simulink model "hw3_mdkhan"  (R2017b)
settings: Solver=ode23tb  StartTime=0.0  StopTime=40  RelTol=1e-3  EnableMultiTasking=on
undefined symbols (not defined in the file): sigbuilder_block
libraries: simulink x1
settings Model: Creator=sampad  LastModifiedBy=khan1
settings DataIOCC: LimitDataPoints=on
settings OptimizationCC: LifeSpan=inf
settings DebuggingCC: AllowSymbolicDim=off  SFUnexpectedBacktrackingDiag=warning  SFNoUnconditionalDefaultTransitionDiag=warning  SFExecutionAtInitializationDiag=none
settings ModelReferenceCC: PropagateSignalLabelsOutOfModel=off
settings CodeAppCC: StateflowObjectComments=on
settings GRTTargetCC: TargetLangStandard=C89/C90 (ANSI)
settings ConfigComp: CovMetricSettings=dw  CovHTMLOptions=-sRT=1 -sVT=0 -aTS=1 -bRG=1 -bTC=1 -hTR=0 -nFC=0 -nFD=1 -scm=1 -bcm=1 -xEv=0 -xEM=0  CovHtmlReporting=on  CovSaveCumulativeToWorkspaceVar=on  CovSaveSingleToWorkspaceVar=on  CovExternalEMLEnable=off

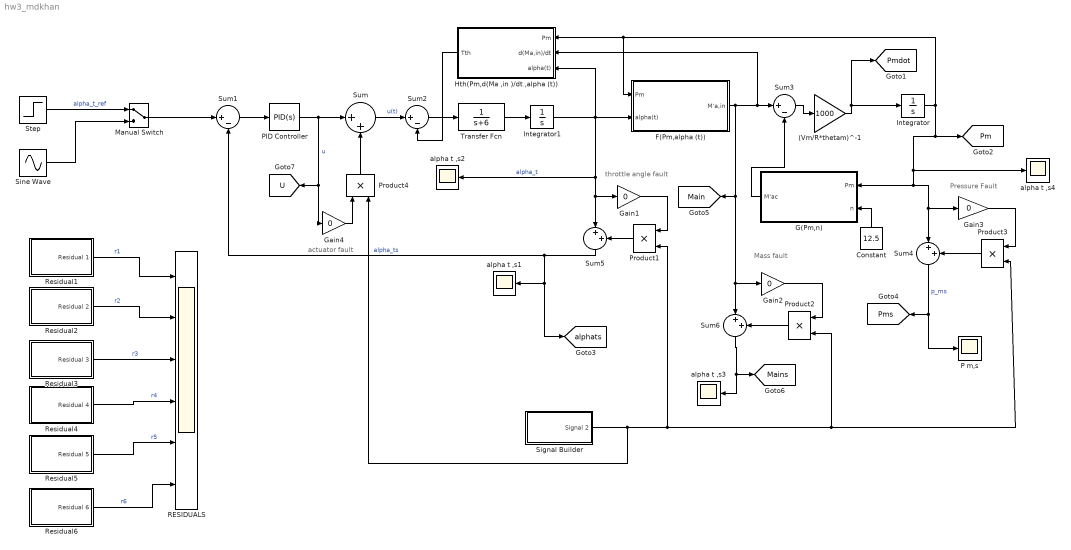
== system hw3_mdkhan ==
  note: actuator fault
  note: throttle angle fault
  note: Mass fault
  note: Pressure Fault
  (Vm/R*thetam)^-1 : Gain  Gain=1000
  Constant : Constant  Value=12.5
  F(Pm,alpha (t)) : Subsystem
  G(Pm,n) : Subsystem
  Gain{1..4} (4 alike) : Gain  Gain=0
  Hth(Pm,d(Ma ,in )/dt ,alpha (t)) : Subsystem
  Integrator : Integrator
  Integrator1 : Integrator
  Manual Switch : ManualSwitch
  P m,s : Scope
  PID Controller : simulink/Continuous/PID Controller  Controller=PID  TimeDomain=Continuous-time  SampleTime=-1  IntegratorMethod=Forward Euler  FilterMethod=Forward Euler  Form=Parallel  UseFilter=on  ControllerParametersSource=internal  P=50.7443606620062  I=163.284224308189  D=3.90171175948325  N=829.275839878731  InitialConditionSource=internal  InitialConditionForIntegrator=0  InitialConditionForFilter=0  ExternalReset=none  LimitOutput=off  UpperSaturationLimit=inf  LowerSaturationLimit=-inf  LinearizeAsGain=on  AntiWindupMode=none  Kb=1  TrackingMode=off  Kt=1  PParamMin=[]  PParamMax=[]  IParamMin=[]  IParamMax=[]  DParamMin=[]  DParamMax=[]  NParamMin=[]  NParamMax=[]  KbParamMin=[]  KbParamMax=[]  KtParamMin=[]  KtParamMax=[]  POutMin=[]  POutMax=[]  IOutMin=[]  IOutMax=[]  DOutMin=[]  DOutMax=[]  NOutMin=[]  NOutMax=[]  KbOutMin=[]  KbOutMax=[]  KtOutMin=[]  KtOutMax=[]  IntegratorOutMin=[]  IntegratorOutMax=[]  FilterOutMin=[]  FilterOutMax=[]  SumOutMin=[]  SumOutMax=[]  SumI1OutMin=[]  SumI1OutMax=[]  SumI2OutMin=[]  SumI2OutMax=[]  SumI3OutMin=[]  SumI3OutMax=[]  SumDOutMin=[]  SumDOutMax=[]  SaturationOutMin=[]  SaturationOutMax=[]  IntegratorContinuousStateAttributes=''  IntegratorStateMustResolveToSignalObject=off  IntegratorRTWStateStorageClass=Auto  FilterContinuousStateAttributes=''  FilterStateMustResolveToSignalObject=off  FilterRTWStateStorageClass=Auto  DifferentiatorICPrevScaledInput=0  DifferentiatorOutMin=[]  DifferentiatorOutMax=[]  InitialConditionSetting=State (most efficient)  FilterDiffOutCoefMin=[]  FilterDiffOutCoefMax=[]  SumDenOutMin=[]  SumDenOutMax=[]  SumNumOutMin=[]  SumNumOutMax=[]  ReciprocalOutMin=[]  ReciprocalOutMax=[]  DivideOutMin=[]  DivideOutMax=[]  TunerSelectOption=Transfer Function Based (PID Tuner App)
  Product{1..4} (4 alike) : Product  RndMeth=Zero
  RESIDUALS : Scope  NumInputPorts=6
  Residual1 : Subsystem
  Residual2 : Subsystem
  Residual3 : Subsystem
  Residual4 : Subsystem
  Residual5 : Subsystem
  Residual6 : Subsystem
  Signal Builder : Subsystem  Tag=STV Subsys  LoadFcn=sigbuilder_block('load');  StartFcn=sigbuilder_block('start');  StopFcn=sigbuilder_block('stop');  ClipboardFcn=sigbuilder_block('clipboard');  mask(Sigbuilder block){tuvar=[0:10]}
      mask help: Create and generate interchangeable groups of signals whose waveforms are piecewise linear.
      mask init:
      | if ~strcmp(get_param(bdroot(gcbh),'SimulationStatus'),'stopped') tuvar = sigbuilder_block('maskInit'); end
      settings: CopyFcn=sigbuilder_block('copy');  DeleteFcn=sigbuilder_block('delete');  ModelCloseFcn=sigbuilder_block('modelClose');  PreSaveFcn=sigbuilder_block('preSave');  PauseFcn=sigbuilder_block('pause')  ContinueFcn=sigbuilder_block('continue')  NameChangeFcn=sigbuilder_block('namechange');  OpenFcn=sigbuilder_block('open',[437.25 117.75 550.5 394.5 ]);  CloseFcn=sigbuilder_block('close');
      mask Display: plot(0, 0, 100, 100,[2, 2, 32, 32, 2], [68, 8, 8, 68, 68],[32, 2], [38, 38], [32, 19, 2],[53, 60, 44], [32, 17, 17, 2],[16, 16, 31, 31]);txt = getActiveGroup(gcbh);text(2, 100, txt,'verticalAlignment', 'top');
  Sine Wave : Sin  SampleTime=0
  Step : Step  Time=0.01  After=20  SampleTime=0
  Sum : Sum  Inputs=|++
  Sum1 : Sum  Inputs=|+-
  Sum2 : Sum  Inputs=|+-
  Sum3 : Sum  Inputs=|+-
  Sum4 : Sum  Inputs=|++  CollapseMode=Specified dimension
  Sum5 : Sum  Inputs=|++  CollapseMode=Specified dimension
  Sum6 : Sum  Inputs=|++  CollapseMode=Specified dimension
  Transfer Fcn : TransferFcn  Denominator=[1 6]
  alpha t ,s{1..4} (4 alike) : Scope
  tag scope: Main=global, Mains=global, Pm=global, Pmdot=global, Pms=global, U=global, alphats=global
  wires:
  Sum1/1 -> PID Controller/1
  PID Controller/1 -> Gain4/1, [U], Sum/1  "u"
  Sum/1 -> Sum2/1  "u(t)"
  Sum2/1 -> Transfer Fcn/1
  Integrator1/1 -> alpha t ,s2/1, Gain1/1, Sum5/1, F(Pm,alpha (t))/2(alpha(t)), Hth(Pm,d(Ma ,in )/dt ,alpha (t))/3(alpha(t))  "alpha_t"
  (Vm/R*thetam)^-1/1 -> Integrator/1, [Pmdot]
  Sum3/1 -> (Vm/R*thetam)^-1/1
  Hth(Pm,d(Ma ,in )/dt ,alpha (t))/1(Tth) -> Sum2/2
  Transfer Fcn/1 -> Integrator1/1
  Product1/1 -> Sum5/2
  Gain1/1 -> Product1/1
  F(Pm,alpha (t))/1(M'a,in) -> [Main], Gain2/1, Sum6/1, Hth(Pm,d(Ma ,in )/dt ,alpha (t))/2(d(Ma,in)/dt), Sum3/1
  Product2/1 -> Sum6/2
  Sum6/1 -> alpha t ,s3/1, [Mains]
  G(Pm,n)/1(M'ac) -> Sum3/2
  Integrator/1 -> F(Pm,alpha (t))/1(Pm), Hth(Pm,d(Ma ,in )/dt ,alpha (t))/1(Pm), alpha t ,s4/1, Gain3/1, Sum4/1, G(Pm,n)/1(Pm), [Pm]
  Product3/1 -> Sum4/2
  Gain3/1 -> Product3/1
  Residual1/1(Residual 1) -> RESIDUALS/1  "r1"
  Residual2/1(Residual 2) -> RESIDUALS/2  "r2"
  Residual3/1(Residual 3) -> RESIDUALS/3  "r3"
  Residual4/1(Residual 4) -> RESIDUALS/4  "r4"
  Residual5/1(Residual 5) -> RESIDUALS/5  "r5"
  Residual6/1(Residual 6) -> RESIDUALS/6  "r6"
  Step/1 -> Manual Switch/1  "alpha_t_ref"
  Manual Switch/1 -> Sum1/1
  Sine Wave/1 -> Manual Switch/2
  Sum5/1 -> [alphats], alpha t ,s1/1, Sum1/2  "alpha_ts"
  Gain2/1 -> Product2/1
  Constant/1 -> G(Pm,n)/2(n)
  Sum4/1 -> P m,s/1, [Pms]  "p_ms"
  Gain4/1 -> Product4/1
  Product4/1 -> Sum/2
  Signal Builder/1(Signal 2) -> Product4/2, Product3/2, Product2/2, Product1/2

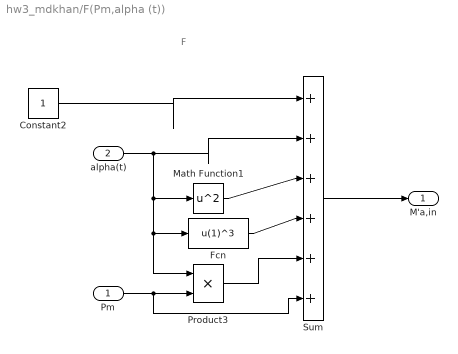
== system hw3_mdkhan/F(Pm,alpha (t)) ==
  note: F
  Pm : Inport
  alpha(t) : Inport  Port=2
  Constant2 : Constant
  Fcn : Fcn  Expr=u(1)^3
  Math Function1 : Math  Operator=square  SaturateOnIntegerOverflow=on
  Product3 : Product  RndMeth=Zero
  Sum : Sum  Inputs=|++++++
  M'a,in : Outport
  wires:
  Sum/1 -> M'a,in/1
  Constant2/1 -> Sum/1
  alpha(t)/1 -> Sum/2, Math Function1/1, Fcn/1, Product3/1
  Math Function1/1 -> Sum/3
  Fcn/1 -> Sum/4
  Product3/1 -> Sum/5
  Pm/1 -> Product3/2, Sum/6

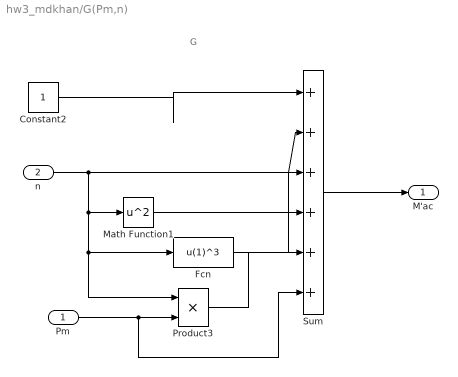
== system hw3_mdkhan/G(Pm,n) ==
  note: G
  Pm : Inport
  n : Inport  Port=2
  Constant2 : Constant
  Fcn : Fcn  Expr=u(1)^3
  Math Function1 : Math  Operator=square  SaturateOnIntegerOverflow=on
  Product3 : Product  RndMeth=Zero
  Sum : Sum  Inputs=|++++++
  M'ac : Outport
  wires:
  Sum/1 -> M'ac/1
  Constant2/1 -> Sum/1
  n/1 -> Sum/2, Math Function1/1, Fcn/1, Product3/1
  Math Function1/1 -> Sum/3
  Fcn/1 -> Sum/4
  Pm/1 -> Product3/2, Sum/6
  Product3/1 -> Sum/5

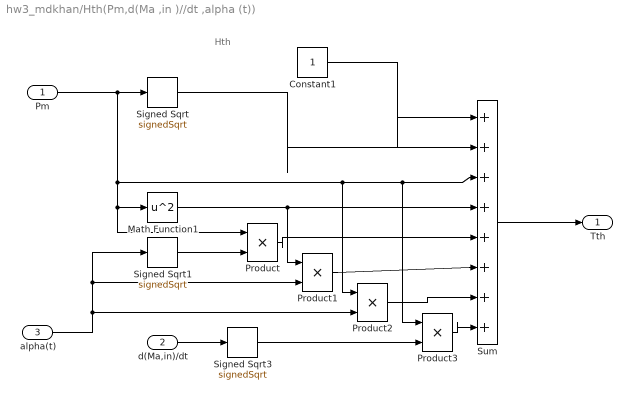
== system hw3_mdkhan/Hth(Pm,d(Ma ,in )//dt ,alpha (t)) ==
  note: Hth
  Pm : Inport
  d(Ma,in)/dt : Inport  Port=2
  alpha(t) : Inport  Port=3
  Constant1 : Constant
  Math Function1 : Math  Operator=square  SaturateOnIntegerOverflow=on
  Product{,1..3} (4 alike) : Product  RndMeth=Zero
  Signed Sqrt : Sqrt  Operator=signedSqrt  SaturateOnIntegerOverflow=on
  Signed Sqrt1 : Sqrt  Operator=signedSqrt  SaturateOnIntegerOverflow=on
  Signed Sqrt3 : Sqrt  Operator=signedSqrt  SaturateOnIntegerOverflow=on
  Sum : Sum  Inputs=|++++++++
  Tth : Outport
  wires:
  Constant1/1 -> Sum/1
  Pm/1 -> Signed Sqrt/1, Math Function1/1, Product/1, Product2/1, Sum/3, Product3/1
  Signed Sqrt/1 -> Sum/2
  Math Function1/1 -> Sum/4, Product1/1
  alpha(t)/1 -> Signed Sqrt1/1, Product1/2, Product2/2
  Signed Sqrt1/1 -> Product/2
  Product/1 -> Sum/5
  Product1/1 -> Sum/6
  Product2/1 -> Sum/7
  Product3/1 -> Sum/8
  d(Ma,in)/dt/1 -> Signed Sqrt3/1
  Signed Sqrt3/1 -> Product3/2
  Sum/1 -> Tth/1

== system hw3_mdkhan/Residual1 ==
  F(Pm,alpha (t)) : Subsystem
  Sum : Sum  Inputs=|+-
  Residual 1 : Outport
  wires:
  [Mains] -> Sum/1
  [Pms] -> F(Pm,alpha (t))/1(Pm)
  [alphats] -> F(Pm,alpha (t))/2(alpha(t))
  F(Pm,alpha (t))/1(M'a,in) -> Sum/2
  Sum/1 -> Residual 1/1

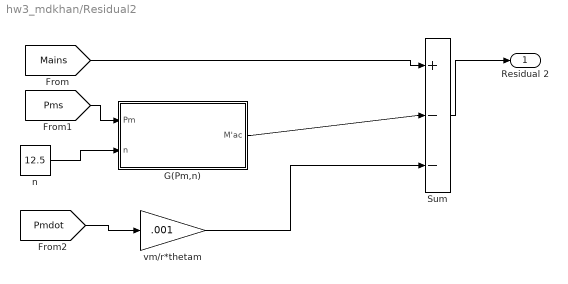
== system hw3_mdkhan/Residual2 ==
  G(Pm,n) : Subsystem
  Sum : Sum  Inputs=|+--
  n : Constant  Value=12.5
  vm/r*thetam : Gain  Gain=.001
  Residual 2 : Outport
  wires:
  Sum/1 -> Residual 2/1
  [Mains] -> Sum/1
  [Pms] -> G(Pm,n)/1(Pm)
  n/1 -> G(Pm,n)/2(n)
  G(Pm,n)/1(M'ac) -> Sum/2
  [Pmdot] -> vm/r*thetam/1
  vm/r*thetam/1 -> Sum/3

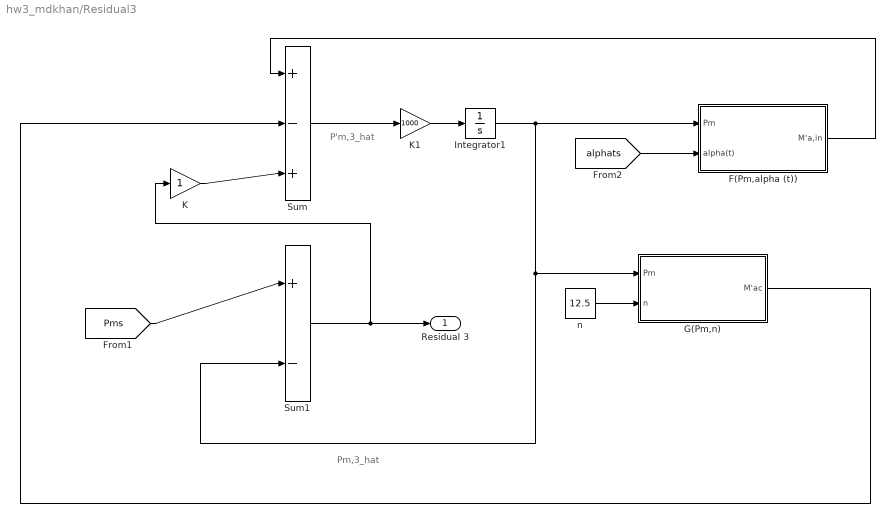
== system hw3_mdkhan/Residual3 ==
  note: Pm,3_hat
  note: P'm,3_hat
  F(Pm,alpha (t)) : Subsystem
  G(Pm,n) : Subsystem
  Integrator1 : Integrator
  K : Gain
  K1 : Gain  Gain=1000
  Sum : Sum  Inputs=|+-+
  Sum1 : Sum  Inputs=|+-
  n : Constant  Value=12.5
  Residual 3 : Outport
  wires:
  [Pms] -> Sum1/1
  K/1 -> Sum/3
  Sum1/1 -> K/1, Residual 3/1
  Sum/1 -> K1/1
  K1/1 -> Integrator1/1
  Integrator1/1 -> F(Pm,alpha (t))/1(Pm), Sum1/2, G(Pm,n)/1(Pm)
  [alphats] -> F(Pm,alpha (t))/2(alpha(t))
  F(Pm,alpha (t))/1(M'a,in) -> Sum/1
  n/1 -> G(Pm,n)/2(n)
  G(Pm,n)/1(M'ac) -> Sum/2

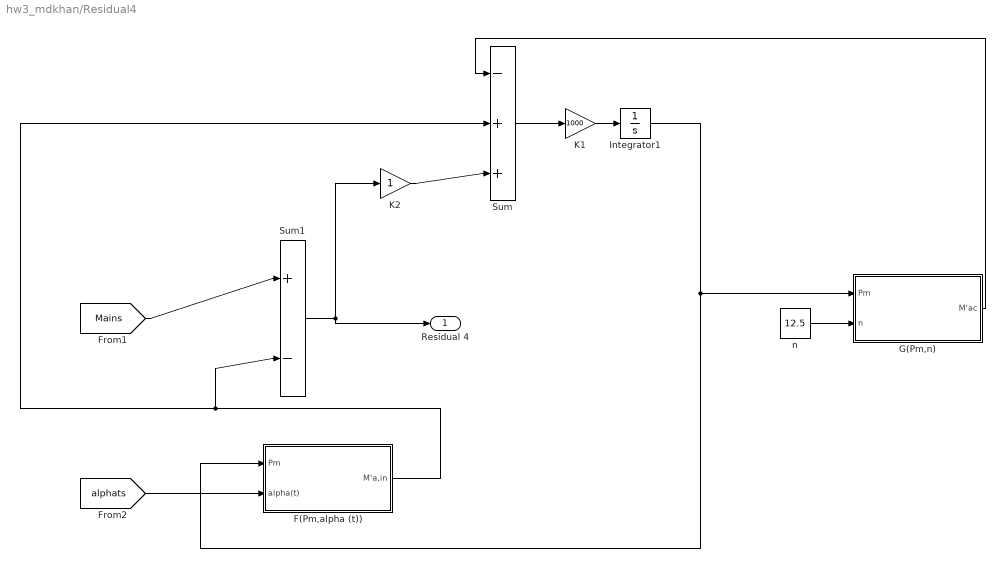
== system hw3_mdkhan/Residual4 ==
  F(Pm,alpha (t)) : Subsystem
  G(Pm,n) : Subsystem
  Integrator1 : Integrator
  K1 : Gain  Gain=1000
  K2 : Gain
  Sum : Sum  Inputs=|-++
  Sum1 : Sum  Inputs=|+-
  n : Constant  Value=12.5
  Residual 4 : Outport
  wires:
  n/1 -> G(Pm,n)/2(n)
  K1/1 -> Integrator1/1
  Sum/1 -> K1/1
  K2/1 -> Sum/3
  [Mains] -> Sum1/1
  [alphats] -> F(Pm,alpha (t))/2(alpha(t))
  Sum1/1 -> Residual 4/1, K2/1
  F(Pm,alpha (t))/1(M'a,in) -> Sum/2, Sum1/2
  Integrator1/1 -> F(Pm,alpha (t))/1(Pm), G(Pm,n)/1(Pm)
  G(Pm,n)/1(M'ac) -> Sum/1

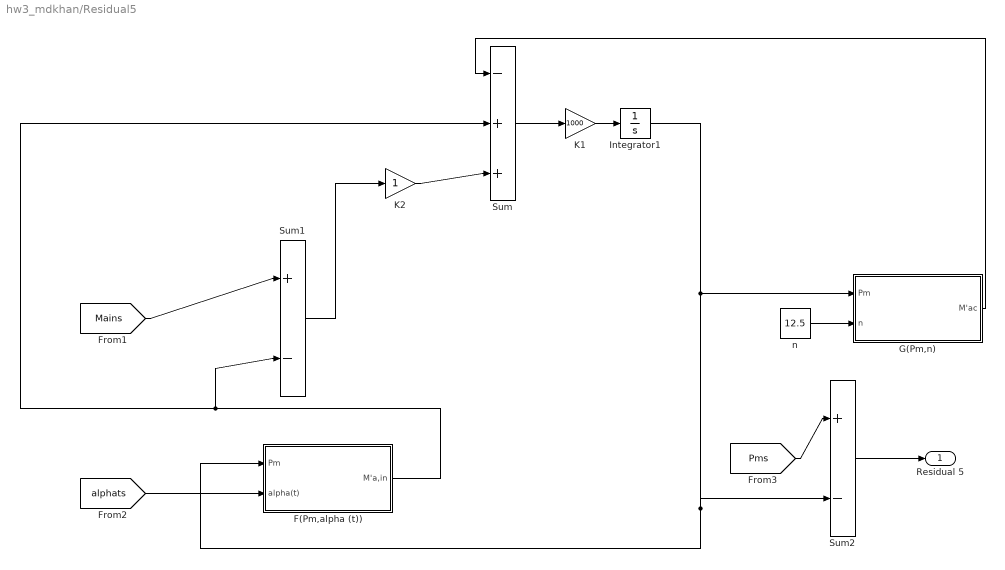
== system hw3_mdkhan/Residual5 ==
  F(Pm,alpha (t)) : Subsystem
  G(Pm,n) : Subsystem
  Integrator1 : Integrator
  K1 : Gain  Gain=1000
  K2 : Gain
  Sum : Sum  Inputs=|-++
  Sum1 : Sum  Inputs=|+-
  Sum2 : Sum  Inputs=|+-
  n : Constant  Value=12.5
  Residual 5 : Outport
  wires:
  G(Pm,n)/1(M'ac) -> Sum/1
  Integrator1/1 -> G(Pm,n)/1(Pm), F(Pm,alpha (t))/1(Pm), Sum2/2
  F(Pm,alpha (t))/1(M'a,in) -> Sum1/2, Sum/2
  Sum1/1 -> K2/1
  [alphats] -> F(Pm,alpha (t))/2(alpha(t))
  [Mains] -> Sum1/1
  K2/1 -> Sum/3
  Sum/1 -> K1/1
  K1/1 -> Integrator1/1
  n/1 -> G(Pm,n)/2(n)
  Sum2/1 -> Residual 5/1
  [Pms] -> Sum2/1

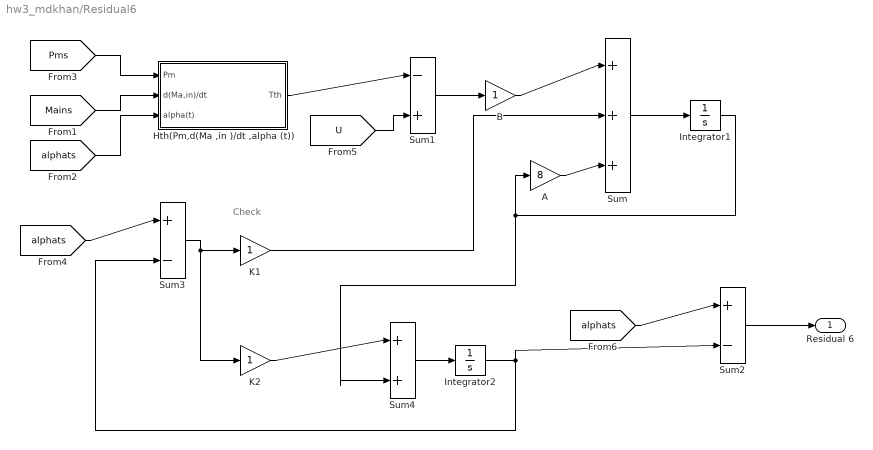
== system hw3_mdkhan/Residual6 ==
  note: Check
  A : Gain  Gain=8
  B : Gain
  Hth(Pm,d(Ma ,in )/dt ,alpha (t)) : Subsystem
  Integrator1 : Integrator
  Integrator2 : Integrator
  K1 : Gain
  K2 : Gain
  Sum : Sum  Inputs=|+++
  Sum1 : Sum  Inputs=|-+
  Sum2 : Sum  Inputs=|+-
  Sum3 : Sum  Inputs=|+-
  Sum4 : Sum  Inputs=|++
  Residual 6 : Outport
  wires:
  [Pms] -> Hth(Pm,d(Ma ,in )/dt ,alpha (t))/1(Pm)
  [Mains] -> Hth(Pm,d(Ma ,in )/dt ,alpha (t))/2(d(Ma,in)/dt)
  [alphats] -> Hth(Pm,d(Ma ,in )/dt ,alpha (t))/3(alpha(t))
  Hth(Pm,d(Ma ,in )/dt ,alpha (t))/1(Tth) -> Sum1/1
  [U] -> Sum1/2
  Sum1/1 -> B/1
  B/1 -> Sum/1
  [alphats] -> Sum3/1
  Sum3/1 -> K1/1, K2/1
  K1/1 -> Sum/2
  Sum/1 -> Integrator1/1
  Integrator1/1 -> A/1, Sum4/2
  A/1 -> Sum/3
  Sum4/1 -> Integrator2/1
  Integrator2/1 -> Sum2/2, Sum3/2
  [alphats] -> Sum2/1
  Sum2/1 -> Residual 6/1
  K2/1 -> Sum4/1

== system hw3_mdkhan/Signal Builder ==
  Demux : Demux  Tag=STV Demux  Outputs=1
  FromWs : FromWorkspace  Tag=STV FromWs  VariableName=tuvar  SampleTime=0
      SigBuilderData=|
      | common.afterFinalStr = 'Extrapolate'
      | common.sampleTime = 0
      | dataSet.timeRange = [0 50]
      | dataSet.name = 'Group 1'
      | sbobj.Groups.Name = 'Group 1'
      | sbobj.Groups.Signals.Name = 'Signal 2'
      | sbobj.Groups.Signals.XData = [0 10 10 30 30 50]
      | sbobj.Groups.Signals.YData = [0 0 1 1 0 0]
      | sbobj.Groups.TimeRange = [0 50]
  Signal 2 : Outport  Tag=STV Outport
  wires:
  FromWs/1 -> Demux/1
  Demux/1 -> Signal 2/1

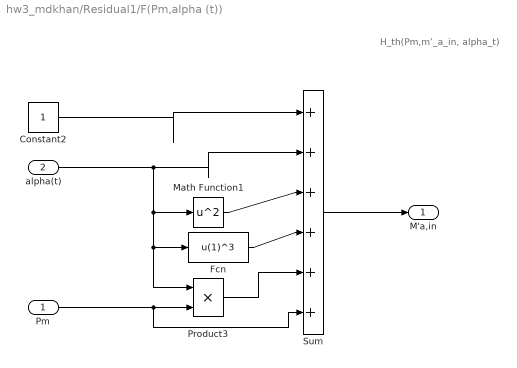
== system hw3_mdkhan/Residual1/F(Pm,alpha (t)) ==
  note: H_th(Pm,m’_a_in, alpha_t)
  Pm : Inport
  alpha(t) : Inport  Port=2
  Constant2 : Constant
  Fcn : Fcn  Expr=u(1)^3
  Math Function1 : Math  Operator=square  SaturateOnIntegerOverflow=on
  Product3 : Product  RndMeth=Zero
  Sum : Sum  Inputs=|++++++
  M'a,in : Outport
  wires:
  Sum/1 -> M'a,in/1
  Constant2/1 -> Sum/1
  alpha(t)/1 -> Sum/2, Math Function1/1, Fcn/1, Product3/1
  Math Function1/1 -> Sum/3
  Fcn/1 -> Sum/4
  Product3/1 -> Sum/5
  Pm/1 -> Product3/2, Sum/6

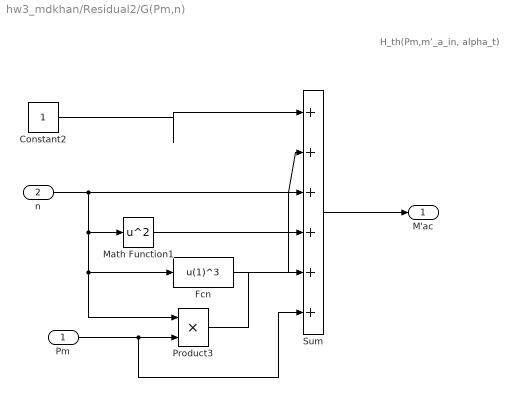
== system hw3_mdkhan/Residual2/G(Pm,n) ==
  note: H_th(Pm,m’_a_in, alpha_t)
  Pm : Inport
  n : Inport  Port=2
  Constant2 : Constant
  Fcn : Fcn  Expr=u(1)^3
  Math Function1 : Math  Operator=square  SaturateOnIntegerOverflow=on
  Product3 : Product  RndMeth=Zero
  Sum : Sum  Inputs=|++++++
  M'ac : Outport
  wires:
  Sum/1 -> M'ac/1
  Constant2/1 -> Sum/1
  n/1 -> Sum/2, Math Function1/1, Fcn/1, Product3/1
  Math Function1/1 -> Sum/3
  Fcn/1 -> Sum/4
  Pm/1 -> Product3/2, Sum/6
  Product3/1 -> Sum/5

== system hw3_mdkhan/Residual3/F(Pm,alpha (t)) ==
  note: H_th(Pm,m’_a_in, alpha_t)
  Pm : Inport
  alpha(t) : Inport  Port=2
  Constant2 : Constant
  Fcn : Fcn  Expr=u(1)^3
  Math Function1 : Math  Operator=square  SaturateOnIntegerOverflow=on
  Product3 : Product  RndMeth=Zero
  Sum : Sum  Inputs=|++++++
  M'a,in : Outport
  wires:
  Sum/1 -> M'a,in/1
  Constant2/1 -> Sum/1
  alpha(t)/1 -> Sum/2, Math Function1/1, Fcn/1, Product3/1
  Math Function1/1 -> Sum/3
  Fcn/1 -> Sum/4
  Product3/1 -> Sum/5
  Pm/1 -> Product3/2, Sum/6

== system hw3_mdkhan/Residual3/G(Pm,n) ==
  note: H_th(Pm,m’_a_in, alpha_t)
  Pm : Inport
  n : Inport  Port=2
  Constant2 : Constant
  Fcn : Fcn  Expr=u(1)^3
  Math Function1 : Math  Operator=square  SaturateOnIntegerOverflow=on
  Product3 : Product  RndMeth=Zero
  Sum : Sum  Inputs=|++++++
  M'ac : Outport
  wires:
  Sum/1 -> M'ac/1
  Constant2/1 -> Sum/1
  n/1 -> Sum/2, Math Function1/1, Fcn/1, Product3/1
  Math Function1/1 -> Sum/3
  Fcn/1 -> Sum/4
  Pm/1 -> Product3/2, Sum/6
  Product3/1 -> Sum/5

== system hw3_mdkhan/Residual4/F(Pm,alpha (t)) ==
  Pm : Inport
  alpha(t) : Inport  Port=2
  Constant2 : Constant
  Fcn : Fcn  Expr=u(1)^3
  Math Function1 : Math  Operator=square  SaturateOnIntegerOverflow=on
  Product3 : Product  RndMeth=Zero
  Sum : Sum  Inputs=|++++++
  M'a,in : Outport
  wires:
  Pm/1 -> Sum/6, Product3/2
  Product3/1 -> Sum/5
  Fcn/1 -> Sum/4
  Math Function1/1 -> Sum/3
  alpha(t)/1 -> Product3/1, Fcn/1, Math Function1/1, Sum/2
  Constant2/1 -> Sum/1
  Sum/1 -> M'a,in/1

== system hw3_mdkhan/Residual4/G(Pm,n) ==
  note: H_th(Pm,m’_a_in, alpha_t)
  Pm : Inport
  n : Inport  Port=2
  Constant2 : Constant
  Fcn : Fcn  Expr=u(1)^3
  Math Function1 : Math  Operator=square  SaturateOnIntegerOverflow=on
  Product3 : Product  RndMeth=Zero
  Sum : Sum  Inputs=|++++++
  M'ac : Outport
  wires:
  Product3/1 -> Sum/5
  Pm/1 -> Sum/6, Product3/2
  Fcn/1 -> Sum/4
  Math Function1/1 -> Sum/3
  n/1 -> Product3/1, Fcn/1, Math Function1/1, Sum/2
  Constant2/1 -> Sum/1
  Sum/1 -> M'ac/1

== system hw3_mdkhan/Residual5/F(Pm,alpha (t)) ==
  note: H_th(Pm,m’_a_in, alpha_t)
  Pm : Inport
  alpha(t) : Inport  Port=2
  Constant2 : Constant
  Fcn : Fcn  Expr=u(1)^3
  Math Function1 : Math  Operator=square  SaturateOnIntegerOverflow=on
  Product3 : Product  RndMeth=Zero
  Sum : Sum  Inputs=|++++++
  M'a,in : Outport
  wires:
  Sum/1 -> M'a,in/1
  Constant2/1 -> Sum/1
  alpha(t)/1 -> Sum/2, Math Function1/1, Fcn/1, Product3/1
  Math Function1/1 -> Sum/3
  Fcn/1 -> Sum/4
  Product3/1 -> Sum/5
  Pm/1 -> Product3/2, Sum/6

== system hw3_mdkhan/Residual5/G(Pm,n) ==
  note: H_th(Pm,m’_a_in, alpha_t)
  Pm : Inport
  n : Inport  Port=2
  Constant2 : Constant
  Fcn : Fcn  Expr=u(1)^3
  Math Function1 : Math  Operator=square  SaturateOnIntegerOverflow=on
  Product3 : Product  RndMeth=Zero
  Sum : Sum  Inputs=|++++++
  M'ac : Outport
  wires:
  Sum/1 -> M'ac/1
  Constant2/1 -> Sum/1
  n/1 -> Sum/2, Math Function1/1, Fcn/1, Product3/1
  Math Function1/1 -> Sum/3
  Fcn/1 -> Sum/4
  Pm/1 -> Product3/2, Sum/6
  Product3/1 -> Sum/5

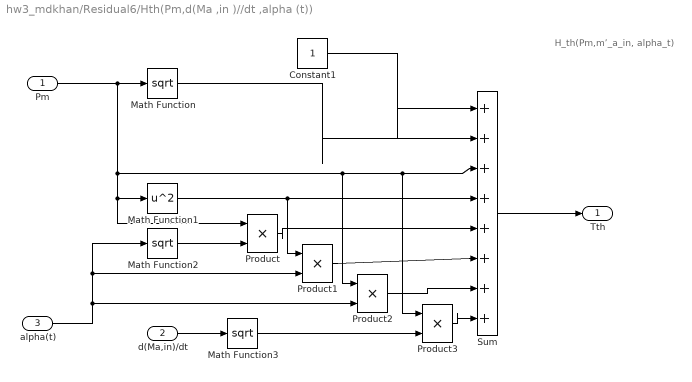
== system hw3_mdkhan/Residual6/Hth(Pm,d(Ma ,in )//dt ,alpha (t)) ==
  note: H_th(Pm,m’_a_in, alpha_t)
  Pm : Inport
  d(Ma,in)/dt : Inport  Port=2
  alpha(t) : Inport  Port=3
  Constant1 : Constant
  Math Function : Math  Operator=sqrt  SaturateOnIntegerOverflow=on
  Math Function1 : Math  Operator=square  SaturateOnIntegerOverflow=on
  Math Function2 : Math  Operator=sqrt  SaturateOnIntegerOverflow=on
  Math Function3 : Math  Operator=sqrt  SaturateOnIntegerOverflow=on
  Product{,1..3} (4 alike) : Product  RndMeth=Zero
  Sum : Sum  Inputs=|++++++++
  Tth : Outport
  wires:
  Constant1/1 -> Sum/1
  Pm/1 -> Math Function/1, Math Function1/1, Product/1, Product2/1, Sum/3, Product3/1
  Math Function/1 -> Sum/2
  Math Function1/1 -> Sum/4, Product1/1
  alpha(t)/1 -> Math Function2/1, Product1/2, Product2/2
  Math Function2/1 -> Product/2
  Product/1 -> Sum/5
  Product1/1 -> Sum/6
  Product2/1 -> Sum/7
  Product3/1 -> Sum/8
  d(Ma,in)/dt/1 -> Math Function3/1
  Math Function3/1 -> Product3/2
  Sum/1 -> Tth/1
